simulink model "PMSM"  (Simulink 8.3)
settings: Solver=ode45  StartTime=0.0  StopTime=1  RelTol=1e-3
undefined symbols (not defined in the file): DiscIntNeverNeededParam
libraries: powerlib_meascontrol x9, powerlib x5
settings Model: Creator=JC  LastModifiedBy=JC
settings DataIOCC: SignalLoggingSaveFormat=Dataset
settings DebuggingCC: UnderspecifiedInitializationDetection=Simplified  StateNameClashWarn=none
settings GRTTargetCC: CombineOutputUpdateFcns=on  GRTInterface=off

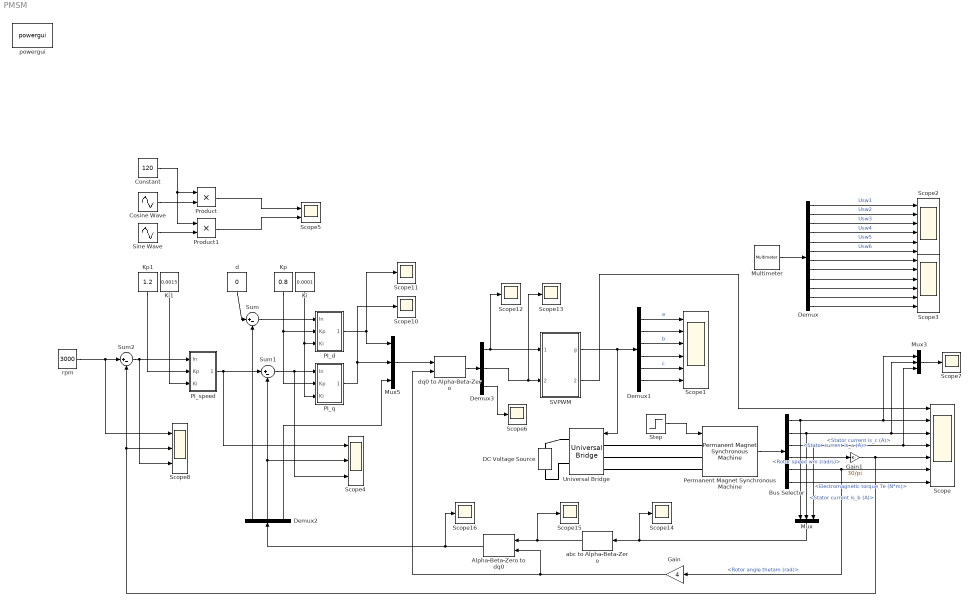
== system PMSM ==
  " Cosine Wave" : Sin  Frequency=pi*2/0.36  Phase=pi/2  Samples=360  SampleTime=0.001  Offset=90
  Alpha-Beta-Zero to dq0 : powerlib_meascontrol/Transformations/Alpha-Beta-Zero to dq0  Alignment=Aligned with phase A axis
  Bus Selector : BusSelector  OutputSignals=Stator current is_a (A),Stator current is_b (A),Stator current is_c (A),Rotor speed wm (rad/s),Rotor angle thetam (rad),Electromagnetic torque Te (N*m)
  Constant : Constant  Value=120
  DC Voltage Source : powerlib/Electrical Sources/DC Voltage Source  Amplitude=310  Measurements=None
  Demux : Demux  Outputs=12
  Demux1 : Demux  Outputs=6
  Demux2 : Demux  Outputs=3
  Demux3 : Demux  Outputs=3
  Gain : Gain  Gain=4
  Gain1 : Gain  Gain=30/pi
  Ki : Constant  Value=0.0001
  Ki1 : Constant  Value=0.0015
  Kp : Constant  Value=0.8
  Kp1 : Constant  Value=1.2
  Multimeter : powerlib/Measurements/Multimeter  PhasorSimulation=off  OutputType=Complex  sel=[1 2 3 4 5 6 11 12 13 14 15 16]  L=16  Gain=[1 1 1 1 1 1 1 1 1 1 1 1]  yselected={'Usw1: Universal Bridge','Usw2: Universal Bridge','Usw3: Universal Bridge','Usw4: Universal Bridge','Usw5: Universal Bridge','Usw6: Universal Bridge','Isw1: Universal Bridge','Isw2: Universal Bridge','Isw3: Universal Bridge','Isw4: Universal Bridge','Isw5: Universal Bridge','Isw6: Universal Bridge'};  PSBOutputType=1  PSBequivalent=0  AxesSetting=[0,0.1,-100,100]  Display=0  SavedBlockNames=-11
  Mux : Mux  Inputs=3
  Mux3 : Mux  Inputs=3
  Mux5 : Mux  Inputs=3
  PI_d : Subsystem
  PI_q : Subsystem
  PI_speed : Subsystem
  Permanent Magnet Synchronous Machine : powerlib/Machines/Permanent Magnet Synchronous Machine  NbPhases=3  FluxDistribution=Sinusoidal  RotorType=Round  MechanicalLoad=Torque Tm  PresetModel=No  ShowDetailedParameters=on  MeasurementBus=off  Resistance=3.3  Inductance=8.5e-3  dqInductances=[8.5e-3,8.5e-3]  La=0.00956  MachineConstant=Flux linkage established by magnets (V.s)  Flux=0.07147  VoltageCst=51.8529  TorqueCst=0.42882  Flat=120  Mechanical=[0.00062 0.0003035 4 0]  PolePairs=4  InitialConditions=[0,0, 0,0]  InitialConditions5ph=[0 0 0 0 0 0]  TsPowergui=0  TsBlock=-1  RefAngle=Aligned with phase A axis (original Park)
  Product : Product
  Product1 : Product
  SVPWM : Subsystem
  Scope : Scope  NumInputPorts=7
      settings: YMin=0~-5~-5~-5~-5~0~-5  YMax=8~5~5~5~5~10~5  SaveName=ScopeData2
  Scope1 : Scope  NumInputPorts=6
      settings: YMin=-5~-5~-5~-5~-5~-5  YMax=5~5~5~5~5~5  SaveName=ScopeData6
  Scope{6..7,10..16} (9 alike) : Scope
      Scope10 settings: SaveName=ScopeData15
      Scope11 settings: SaveName=ScopeData16
      Scope12 settings: SaveName=ScopeData17
      Scope13 settings: SaveName=ScopeData18
      Scope14 settings: SaveName=ScopeData19
      Scope15 settings: SaveName=ScopeData20
      Scope16 settings: SaveName=ScopeData21
      Scope6 settings: SaveName=ScopeData11
      Scope7 settings: SaveName=ScopeData12
  Scope2 : Scope  NumInputPorts=6
      settings: YMin=-5~-5~-5~-5~-5~-5  YMax=5~5~5~5~5~5
  Scope3 : Scope  NumInputPorts=6
      settings: YMin=-5~-5~-5~-5~-5~-5  YMax=5~5~5~5~5~5  SaveName=ScopeData8
  Scope4 : Scope  NumInputPorts=3
      settings: YMin=-5~-5~-5  YMax=5~5~5  SaveName=ScopeData9
  Scope5 : Scope  NumInputPorts=2
      settings: YMin=-5~-5  YMax=5~5  SaveName=ScopeData10
  Scope8 : Scope  NumInputPorts=3
      settings: YMin=-5~-5~-5  YMax=5~5~5  SaveName=ScopeData13
  Sine Wave : Sin  Frequency=pi*2/0.36  Samples=360  SampleTime=0.001
  Step : Step  Time=0  After=0  SampleTime=0
  Sum : Sum  Inputs=|+-
  Sum1 : Sum  Inputs=|+-
  Sum2 : Sum  Inputs=|+-
  Universal Bridge : powerlib/Power Electronics/Universal Bridge  Arms=3  SnubberResistance=1e5  SnubberCapacitance=inf  Device=IGBT / Diodes  Ron=1e-3  Lon=0  ForwardVoltages="[  0  0  ]"  ForwardVoltage=0  GTOparameters=[ 10e-6 , 20e-6 ]  IGBTparameters=[ 1e-6 , 2e-6 ]  Measurements=All voltages and currents  Measurements_2=None  converterType=Rectifier
  abc to Alpha-Beta-Zero : powerlib_meascontrol/Transformations/abc to Alpha-Beta-Zero
  d : Constant  Value=0
  dq0 to Alpha-Beta-Zero : powerlib_meascontrol/Transformations/dq0 to Alpha-Beta-Zero  Alignment=Aligned with phase A axis
  powergui : powerlib/powergui  RequirementInfo="{}  %GIDa_c9ce1342_5d33_47b2_941f_a20f6faa6b6c"  Priority=1  SimulationMode=Discrete  SolverType=Tustin  SampleTime=50e-6  frequency=60  SPID=off  DisableSnubberDevices=off  DisableRonSwitches=off  DisableVfSwitches=off  SwTol=0  Interpol=off  DisplayEquations=off  Ts=0  methode=off  frequencyindice=0  Pbase=100e6  ErrMax=1e-4  Iterations=50  UnitsV=kV  UnitsW=MW  FunctionMessages=off  echomessages=off  HookPort=off  EnableUseOfTLC=off  x0status=blocks  RestoreLinks=warning  ResistiveCurrentMeasurement=off  Frange=[0:2:500]  Ylog=off  Xlog=on  ShowGrid=off  save=off  variable=ZData  structure=0  ZoomFFT=off  StartTime=0.0  cycles=1  DisplayStyle=1  fundamental=60  FreqAxis=off  MaxFrequency=1000  frequencyindicesteady=1  RmsSteady=1  display=off
  rpm : Constant  Value=3000
  wires:
  Step/1 -> Permanent Magnet Synchronous Machine/1
  Bus Selector/2 -> Mux3/2, Scope/3, Mux/2  "<Stator current is_b (A)>"
  Bus Selector/3 -> Mux3/3, Scope/4, Mux/3  "<Stator current is_c (A)>"
  Bus Selector/4 -> Gain1/1  "<Rotor speed wm (rad/s)>"
  Bus Selector/5 -> Gain/1, Scope/6  "<Rotor angle thetam (rad)>"
  Bus Selector/6 -> Scope/7  "<Electromagnetic torque Te (N*m)>"
  Multimeter/1 -> Demux/1
  SVPWM/1(g) -> Demux1/1, Universal Bridge/1
  Demux1/1 -> Scope1/1  "a"
  Demux1/2 -> Scope1/2
  Demux1/3 -> Scope1/3  "b"
  Demux1/4 -> Scope1/4
  Demux1/5 -> Scope1/5  "c"
  Demux1/6 -> Scope1/6
  SVPWM/2(sector) -> Scope/1
  Bus Selector/1 -> Mux3/1, Scope/2, Mux/1  "<Stator current is_a (A)>"
  Permanent Magnet Synchronous Machine/1 -> Bus Selector/1
  abc to Alpha-Beta-Zero/1 -> Scope15/1, Alpha-Beta-Zero to dq0/1
  Constant/1 -> Product1/1, Product/1
  " Cosine Wave"/1 -> Product/2
  Sine Wave/1 -> Product1/2
  Product/1 -> Scope5/1
  Product1/1 -> Scope5/2
  dq0 to Alpha-Beta-Zero/1 -> Demux3/1
  Demux3/3 -> Scope6/1
  Demux3/1 -> SVPWM/1(Ualpha), Scope12/1
  Demux3/2 -> Scope13/1, SVPWM/2("Ubeta ")
  Mux3/1 -> Scope7/1
  Alpha-Beta-Zero to dq0/1 -> Scope16/1, Demux2/1
  Mux/1 -> Scope14/1, abc to Alpha-Beta-Zero/1
  Gain/1 -> dq0 to Alpha-Beta-Zero/2, Alpha-Beta-Zero to dq0/2
  Demux2/1 -> Sum/2
  Sum/1 -> PI_d/1(In)
  Demux2/2 -> Sum1/2, Scope4/2
  Sum1/1 -> Scope4/3, PI_q/1(In)
  PI_q/1("Out ") -> Mux5/2, Scope10/1
  PI_d/1("Out ") -> Scope11/1, Mux5/1
  Mux5/1 -> dq0 to Alpha-Beta-Zero/1
  d/1 -> Sum/1
  PI_speed/1("Out ") -> Scope4/1, Sum1/1
  Ki/1 -> PI_d/3(Ki), PI_q/3(Ki)
  Kp/1 -> PI_d/2(Kp), PI_q/2(Kp)
  Demux2/3 -> Mux5/3
  Gain1/1 -> Scope/5, Sum2/2, Scope8/2
  Ki1/1 -> PI_speed/3(Ki)
  Kp1/1 -> PI_speed/2(Kp)
  Sum2/1 -> Scope8/3, PI_speed/1(In)
  rpm/1 -> Scope8/1, Sum2/1
  Demux/1 -> Scope2/1  "Usw1"
  Demux/2 -> Scope2/2  "Usw2"
  Demux/3 -> Scope2/3  "Usw3"
  Demux/4 -> Scope2/4  "Usw4"
  Demux/5 -> Scope2/5  "Usw5"
  Demux/6 -> Scope2/6  "Usw6"
  Demux/7 -> Scope3/1
  Demux/8 -> Scope3/2
  Demux/9 -> Scope3/3
  Demux/10 -> Scope3/4
  Demux/11 -> Scope3/5
  Demux/12 -> Scope3/6
  connections:
  Universal Bridge/LConn1 -- Permanent Magnet Synchronous Machine/LConn1
  Universal Bridge/LConn2 -- Permanent Magnet Synchronous Machine/LConn2
  Universal Bridge/LConn3 -- Permanent Magnet Synchronous Machine/LConn3
  Universal Bridge/RConn1 -- DC Voltage Source/RConn1
  Universal Bridge/RConn2 -- DC Voltage Source/LConn1

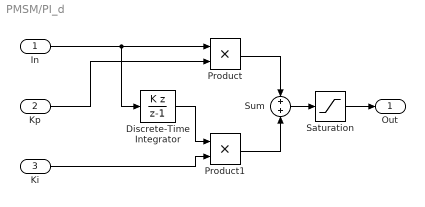
== system PMSM/PI_d ==
  In : Inport
  Kp : Inport  Port=2
  Ki : Inport  Port=3
  Discrete-Time Integrator : DiscreteIntegrator  IntegratorMethod=Accumulation: Backward Euler  SampleTime=0.0005  ICPrevOutput=DiscIntNeverNeededParam  ICPrevScaledInput=DiscIntNeverNeededParam
  Product : Product
  Product1 : Product
  Saturation : Saturate  UpperLimit=300  LowerLimit=-300
  Sum : Sum  Inputs=+|+
  "Out " : Outport
  wires:
  In/1 -> Discrete-Time Integrator/1, Product/1
  Kp/1 -> Product/2
  Discrete-Time Integrator/1 -> Product1/1
  Ki/1 -> Product1/2
  Product/1 -> Sum/1
  Product1/1 -> Sum/2
  Sum/1 -> Saturation/1
  Saturation/1 -> "Out "/1

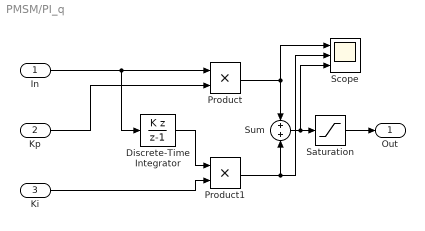
== system PMSM/PI_q ==
  In : Inport
  Kp : Inport  Port=2
  Ki : Inport  Port=3
  Discrete-Time Integrator : DiscreteIntegrator  IntegratorMethod=Accumulation: Backward Euler  SampleTime=0.0005  ICPrevOutput=DiscIntNeverNeededParam  ICPrevScaledInput=DiscIntNeverNeededParam
  Product : Product
  Product1 : Product
  Saturation : Saturate  UpperLimit=300  LowerLimit=-300
  Scope : Scope  NumInputPorts=3
      settings: YMin=-5~-5~-5  YMax=5~5~5  SaveName=ScopeData22
  Sum : Sum  Inputs=+|+
  "Out " : Outport
  wires:
  In/1 -> Discrete-Time Integrator/1, Product/1
  Kp/1 -> Product/2
  Discrete-Time Integrator/1 -> Product1/1
  Ki/1 -> Product1/2
  Product/1 -> Scope/1, Sum/1
  Product1/1 -> Sum/2, Scope/2
  Sum/1 -> Scope/3, Saturation/1
  Saturation/1 -> "Out "/1

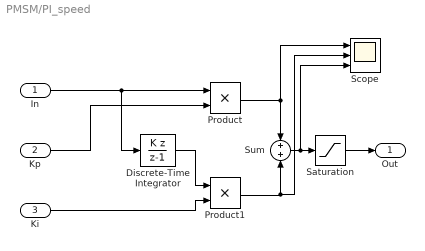
== system PMSM/PI_speed ==
  In : Inport
  Kp : Inport  Port=2
  Ki : Inport  Port=3
  Discrete-Time Integrator : DiscreteIntegrator  IntegratorMethod=Accumulation: Backward Euler  SampleTime=0.0005  ICPrevOutput=DiscIntNeverNeededParam  ICPrevScaledInput=DiscIntNeverNeededParam
  Product : Product
  Product1 : Product
  Saturation : Saturate  UpperLimit=4000  LowerLimit=-4000
  Scope : Scope  NumInputPorts=3
      settings: YMin=-5~-5~-5  YMax=5~5~5  SaveName=ScopeData14
  Sum : Sum  Inputs=+|+
  "Out " : Outport
  wires:
  In/1 -> Discrete-Time Integrator/1, Product/1
  Kp/1 -> Product/2
  Discrete-Time Integrator/1 -> Product1/1
  Ki/1 -> Product1/2
  Product/1 -> Sum/1, Scope/1
  Product1/1 -> Scope/2, Sum/2
  Sum/1 -> Scope/3, Saturation/1
  Saturation/1 -> "Out "/1

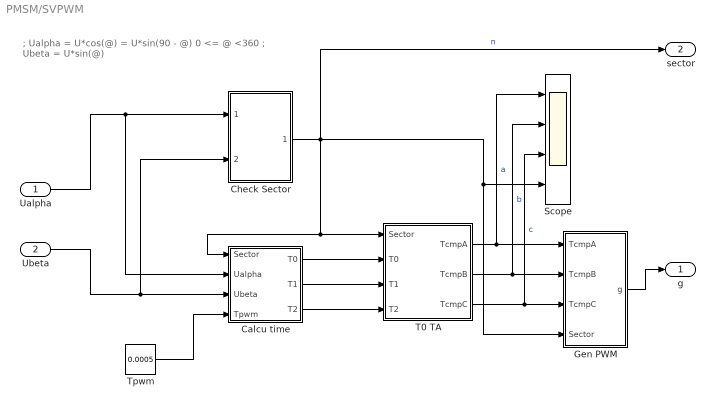
== system PMSM/SVPWM ==
  note: ; Ualpha = U*cos(@) = U*sin(90 - @)  0 <= @ <360
      | ; Ubeta  = U*sin(@)
  Ualpha : Inport
  "Ubeta " : Inport  Port=2
  Calcu time : Subsystem
  Check Sector : Subsystem
  "Gen PWM " : Subsystem
  Scope : Scope  NumInputPorts=4
      settings: YMin=-5~-5~-5~-5  YMax=5~5~5~5  SaveName=ScopeData5
  "T0 TA " : Subsystem
  Tpwm : Constant  Value=0.0005
  g : Outport
  sector : Outport  Port=2
  wires:
  "T0 TA "/1(TcmpA) -> "Gen PWM "/1(TcmpA), Scope/1  "a"
  "T0 TA "/2(TcmpB) -> Scope/2, "Gen PWM "/2(TcmpB)  "b"
  "T0 TA "/3(TcmpC) -> Scope/3, "Gen PWM "/3(TcmpC)  "c"
  Ualpha/1 -> Check Sector/1(Ualpha), Calcu time/2("Ualpha ")
  "Ubeta "/1 -> Check Sector/2(Ubeta), Calcu time/3(Ubeta)
  Check Sector/1(Sector) -> sector/1, Calcu time/1(Sector), "T0 TA "/1(Sector), "Gen PWM "/4(Sector), Scope/4  "n"
  Calcu time/1(T0) -> "T0 TA "/2(T0)
  Calcu time/2(T1) -> "T0 TA "/3(T1)
  Calcu time/3(T2) -> "T0 TA "/4(T2)
  "Gen PWM "/1(g) -> g/1
  Tpwm/1 -> Calcu time/4(Tpwm)

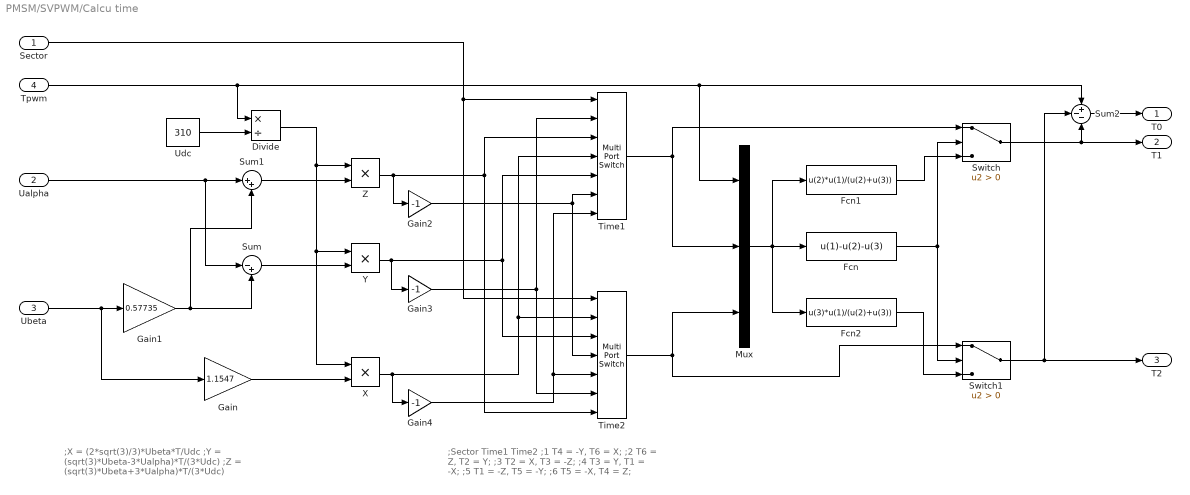
== system PMSM/SVPWM/Calcu time ==
  note: ;Sector	Time1	 Time2
      | ;1	T4 = -Y,	T6 =  X;
      | ;2	T6 =  Z,	T2 =  Y;
      | ;3	T2 =  X,	T3 = -Z;
      | ;4	T3 =  Y,	T1 = -X;
      | ;5	T1 = -Z,	T5 = -Y;
      | ;6	T5 = -X,	T4 =  Z;
  note: ;X = (2*sqrt(3)/3)*Ubeta*T/Udc
      | ;Y = (sqrt(3)*Ubeta-3*Ualpha)*T/(3*Udc)
      | ;Z = (sqrt(3)*Ubeta+3*Ualpha)*T/(3*Udc)
  Sector : Inport
  "Ualpha " : Inport  Port=2
  Ubeta : Inport  Port=3
  Tpwm : Inport  Port=4
  Divide : Product  Inputs=*/
  Fcn : Fcn  Expr=u(1)-u(2)-u(3)
  Fcn1 : Fcn  Expr=u(2)*u(1)/(u(2)+u(3))
  Fcn2 : Fcn  Expr=u(3)*u(1)/(u(2)+u(3))
  Gain : Gain  Gain=1.1547
  Gain1 : Gain  Gain=0.57735
  Gain2 : Gain  Gain=-1
  Gain3 : Gain  Gain=-1
  Gain4 : Gain  Gain=-1
  Mux : Mux  Inputs=3
  Sum : Sum  Inputs=|-+
  Sum1 : Sum  Inputs=|++
  Sum2 : Sum  Inputs=+--
  Switch : Switch  Criteria=u2 > Threshold
  Switch1 : Switch  Criteria=u2 > Threshold
  Time1 : MultiPortSwitch  Inputs=6
  Time2 : MultiPortSwitch  Inputs=6
  Udc : Constant  Value=310
  X : Product
  Y : Product
  Z : Product
  T0 : Outport
  T1 : Outport  Port=2
  T2 : Outport  Port=3
  wires:
  Sum1/1 -> Z/2
  Divide/1 -> X/1, Y/1, Z/1
  Tpwm/1 -> Divide/1, Sum2/1, Mux/1
  Sum/1 -> Y/2
  Gain2/1 -> Time2/4, Time1/6
  Fcn/1 -> Switch1/2, Switch/2
  Time2/1 -> Switch1/1, Mux/3
  Time1/1 -> Mux/2, Switch/1
  Mux/1 -> Fcn2/1, Fcn1/1, Fcn/1
  Y/1 -> Gain3/1, Time2/3, Time1/5
  Gain3/1 -> Time2/6, Time1/2
  Sector/1 -> Time1/1, Time2/1
  Z/1 -> Time1/3, Time2/7, Gain2/1
  Switch1/1 -> T2/1, Sum2/2
  Gain/1 -> X/2
  Switch/1 -> T1/1, Sum2/3
  Udc/1 -> Divide/2
  Gain4/1 -> Time1/7, Time2/5
  Fcn1/1 -> Switch/3
  X/1 -> Time2/2, Time1/4, Gain4/1
  Fcn2/1 -> Switch1/3
  Sum2/1 -> T0/1
  Gain1/1 -> Sum1/2, Sum/2
  Ubeta/1 -> Gain/1, Gain1/1
  "Ualpha "/1 -> Sum/1, Sum1/1

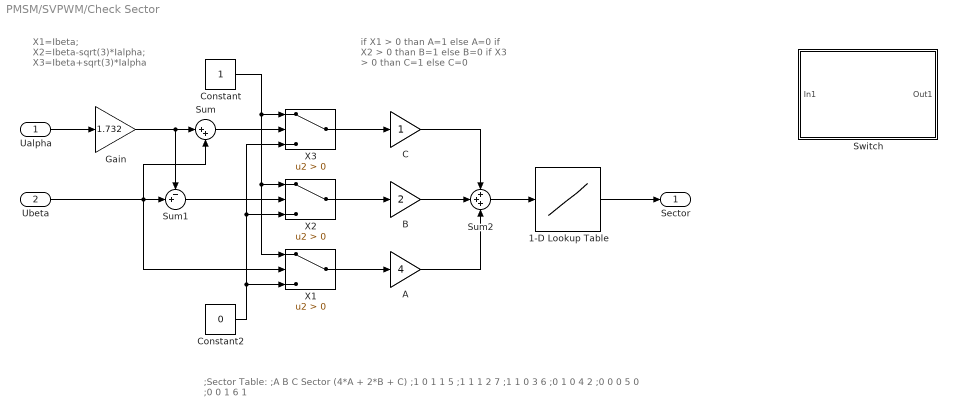
== system PMSM/SVPWM/Check Sector ==
  note: ;Sector Table:
      | ;A	B	C	Sector	(4*A + 2*B + C)
      | ;1	0	1	1	5
      | ;1	1	1	2	7
      | ;1	1	0	3	6
      | ;0	1	0	4	2
      | ;0	0	0	5	0
      | ;0	0	1	6	1
  note: if X1 > 0 than A=1 else A=0
      | if X2 > 0 than B=1 else B=0
      | if X3 > 0 than C=1 else C=0
  note: X1=Ibeta;
      | X2=Ibeta-sqrt(3)*Ialpha;
      | X3=Ibeta+sqrt(3)*Ialpha
  Ualpha : Inport
  Ubeta : Inport  Port=2
  1-D Lookup Table : Lookup_n-D  NumberOfTableDimensions=1  BreakpointsForDimension1=[0 1 2 5 6 7]  Table=[5 6 4 1 3 2]  InternalRulePriority=Speed  RndMeth=Simplest  InputSameDT=on
  A : Gain  Gain=4
  B : Gain  Gain=2
  C : Gain
  Constant : Constant
  Constant2 : Constant  Value=0
  Gain : Gain  Gain=1.732
  Sum : Sum  Inputs=|++
  Sum1 : Sum  Inputs=-+|
  Sum2 : Sum  Inputs=+++
  Switch : Subsystem
  X1 : Switch  Criteria=u2 > Threshold
  X2 : Switch  Criteria=u2 > Threshold
  X3 : Switch  Criteria=u2 > Threshold
  Sector : Outport
  wires:
  Ubeta/1 -> Sum1/2, X1/2, Sum/2
  Gain/1 -> Sum/1, Sum1/1
  Ualpha/1 -> Gain/1
  Sum/1 -> X3/2
  X2/1 -> B/1
  X3/1 -> C/1
  X1/1 -> A/1
  Sum1/1 -> X2/2
  Constant/1 -> X1/1, X2/1, X3/1
  Constant2/1 -> X3/3, X2/3, X1/3
  C/1 -> Sum2/1
  B/1 -> Sum2/2
  A/1 -> Sum2/3
  Sum2/1 -> 1-D Lookup Table/1
  1-D Lookup Table/1 -> Sector/1

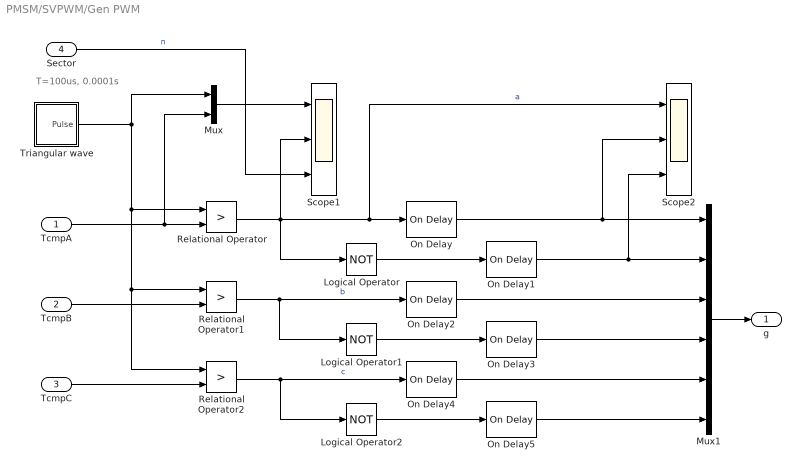
== system PMSM/SVPWM/Gen PWM  ==
  note: T=100us, 0.0001s
  TcmpA : Inport
  TcmpB : Inport  Port=2
  TcmpC : Inport  Port=3
  Sector : Inport  Port=4
  Logical Operator : Logic  Operator=NOT  AllPortsSameDT=off  OutDataTypeStr=boolean
  Logical Operator1 : Logic  Operator=NOT  AllPortsSameDT=off  OutDataTypeStr=boolean
  Logical Operator2 : Logic  Operator=NOT  AllPortsSameDT=off  OutDataTypeStr=boolean
  Mux : Mux  Inputs=2
  Mux1 : Mux  Inputs=6
  On Delay{,1..5} (6 alike) : powerlib_meascontrol/Logic/On Delay  DelayType=On delay  delay=0.000005  ic=0  Ts=0
  Relational Operator : RelationalOperator  Operator=>  OutDataTypeStr=boolean
  Relational Operator1 : RelationalOperator  Operator=>  OutDataTypeStr=boolean
  Relational Operator2 : RelationalOperator  Operator=>  OutDataTypeStr=boolean
  Scope1 : Scope  NumInputPorts=3
      settings: YMin=-5~-5~-5  YMax=5~5~5  SaveName=ScopeData3
  Scope2 : Scope  NumInputPorts=3
      settings: YMin=-5~-5~-5  YMax=5~5~5
  Triangular wave : Subsystem
  g : Outport
  wires:
  Triangular wave/1("Pulse ") -> Relational Operator2/1, Relational Operator1/1, Relational Operator/1, Mux/1
  TcmpA/1 -> Mux/2, Relational Operator/2
  Relational Operator/1 -> Scope1/2, Logical Operator/1, Scope2/1, On Delay/1  "a"
  TcmpB/1 -> Relational Operator1/2
  TcmpC/1 -> Relational Operator2/2
  Relational Operator2/1 -> Logical Operator2/1, On Delay4/1  "c"
  Relational Operator1/1 -> Logical Operator1/1, On Delay2/1  "b"
  Logical Operator2/1 -> On Delay5/1
  Logical Operator1/1 -> On Delay3/1
  Logical Operator/1 -> On Delay1/1
  Mux/1 -> Scope1/1
  Sector/1 -> Scope1/3  "n"
  Mux1/1 -> g/1
  On Delay/1 -> Scope2/2, Mux1/1
  On Delay1/1 -> Scope2/3, Mux1/2
  On Delay2/1 -> Mux1/3
  On Delay3/1 -> Mux1/4
  On Delay4/1 -> Mux1/5
  On Delay5/1 -> Mux1/6

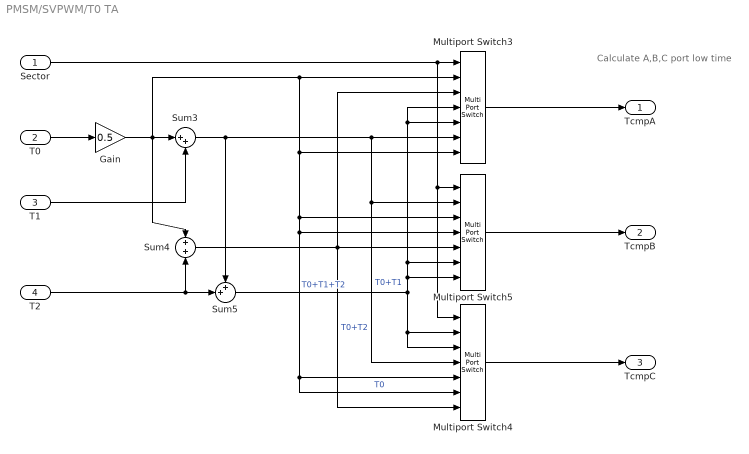
== system PMSM/SVPWM/T0 TA  ==
  note: Calculate A,B,C port low time
  Sector : Inport
  T0 : Inport  Port=2
  T1 : Inport  Port=3
  T2 : Inport  Port=4
  Gain : Gain  Gain=0.5
  Multiport Switch3 : MultiPortSwitch  Inputs=6
  Multiport Switch4 : MultiPortSwitch  Inputs=6
  Multiport Switch5 : MultiPortSwitch  Inputs=6
  Sum3 : Sum  Inputs=|++
  Sum4 : Sum  Inputs=+|+
  Sum5 : Sum  Inputs=++|
  TcmpA : Outport
  TcmpB : Outport  Port=2
  TcmpC : Outport  Port=3
  wires:
  Gain/1 -> Sum4/1, Multiport Switch3/2, Multiport Switch3/7, Multiport Switch4/6, Multiport Switch4/5, Multiport Switch5/4, Multiport Switch5/3, Sum3/1  "T0"
  Sector/1 -> Multiport Switch3/1, Multiport Switch4/1, Multiport Switch5/1
  T0/1 -> Gain/1
  Sum3/1 -> Sum5/1, Multiport Switch4/4, Multiport Switch5/2, Multiport Switch3/6  "T0+T1"
  Sum5/1 -> Multiport Switch5/7, Multiport Switch5/6, Multiport Switch3/5, Multiport Switch3/4, Multiport Switch4/2, Multiport Switch4/3  "T0+T1+T2"
  T1/1 -> Sum3/2
  T2/1 -> Sum5/2, Sum4/2
  Multiport Switch4/1 -> TcmpC/1
  Multiport Switch3/1 -> TcmpA/1
  Multiport Switch5/1 -> TcmpB/1
  Sum4/1 -> Multiport Switch4/7, Multiport Switch5/5, Multiport Switch3/3  "T0+T2"

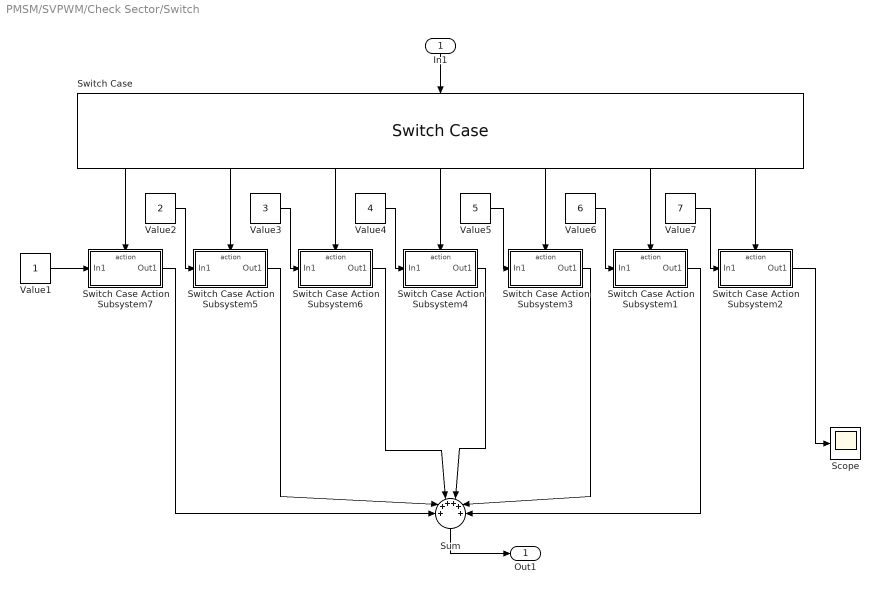
== system PMSM/SVPWM/Check Sector/Switch ==
  In1 : Inport
  Scope : Scope
      settings: SaveName=ScopeData7
  Sum : Sum  Inputs=++++++
  Switch Case : SwitchCase  CaseConditions={5,7,6,2,0,1}
  Switch Case Action Subsystem1 : Subsystem  TreatAsAtomicUnit=on
  Switch Case Action Subsystem2 : Subsystem  TreatAsAtomicUnit=on
  Switch Case Action Subsystem3 : Subsystem  TreatAsAtomicUnit=on
  Switch Case Action Subsystem4 : Subsystem  TreatAsAtomicUnit=on
  Switch Case Action Subsystem5 : Subsystem  TreatAsAtomicUnit=on
  Switch Case Action Subsystem6 : Subsystem  TreatAsAtomicUnit=on
  Switch Case Action Subsystem7 : Subsystem  TreatAsAtomicUnit=on
  Value1 : Constant
  Value2 : Constant  Value=2
  Value3 : Constant  Value=3
  Value4 : Constant  Value=4
  Value5 : Constant  Value=5
  Value6 : Constant  Value=6
  Value7 : Constant  Value=7
  Out1 : Outport
  wires:
  Switch Case Action Subsystem6/1(Out1) -> Sum/3
  Switch Case Action Subsystem3/1(Out1) -> Sum/5
  Switch Case Action Subsystem2/1(Out1) -> Scope/1
  Switch Case Action Subsystem5/1(Out1) -> Sum/2
  Switch Case Action Subsystem1/1(Out1) -> Sum/6
  Switch Case Action Subsystem4/1(Out1) -> Sum/4
  Value6/1 -> Switch Case Action Subsystem1/1(In1)
  Switch Case/5 -> Switch Case Action Subsystem3/Action
  Value1/1 -> Switch Case Action Subsystem7/1(In1)
  Switch Case/3 -> Switch Case Action Subsystem6/Action
  Switch Case/1 -> Switch Case Action Subsystem7/Action
  Switch Case/2 -> Switch Case Action Subsystem5/Action
  Switch Case Action Subsystem7/1(Out1) -> Sum/1
  Switch Case/7 -> Switch Case Action Subsystem2/Action
  Value3/1 -> Switch Case Action Subsystem6/1(In1)
  Value5/1 -> Switch Case Action Subsystem3/1(In1)
  Value7/1 -> Switch Case Action Subsystem2/1(In1)
  Value4/1 -> Switch Case Action Subsystem4/1(In1)
  Switch Case/4 -> Switch Case Action Subsystem4/Action
  Value2/1 -> Switch Case Action Subsystem5/1(In1)
  Switch Case/6 -> Switch Case Action Subsystem1/Action
  Sum/1 -> Out1/1
  In1/1 -> Switch Case/1

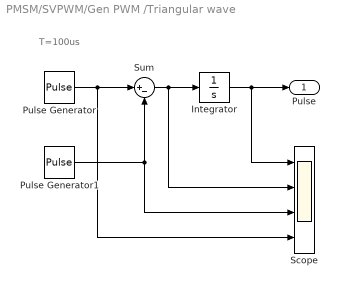
== system PMSM/SVPWM/Gen PWM /Triangular wave ==
  note: T=100us
  Integrator : Integrator
  Pulse Generator : DiscretePulseGenerator  PulseType=Time based  Amplitude=2  Period=0.0005  PulseWidth=50
  Pulse Generator1 : DiscretePulseGenerator  PulseType=Time based  Amplitude=2  Period=0.0005  PulseWidth=50  PhaseDelay=0.00025
  Scope : Scope  NumInputPorts=4
      settings: YMin=-5~-5~-5~-5  YMax=5~5~5~5  SaveName=ScopeData4
  Sum : Sum  Inputs=|+-
  "Pulse " : Outport
  wires:
  Sum/1 -> Scope/2, Integrator/1
  Pulse Generator1/1 -> Scope/3, Sum/2
  Pulse Generator/1 -> Scope/4, Sum/1
  Integrator/1 -> Scope/1, "Pulse "/1

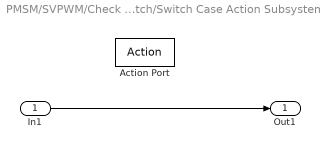
== system PMSM/SVPWM/Check Sector/Switch/Switch Case Action Subsystem1 ==
  In1 : Inport
  Action Port : ActionPort  ActionType=case
  Out1 : Outport
  wires:
  In1/1 -> Out1/1

== system PMSM/SVPWM/Check Sector/Switch/Switch Case Action Subsystem2 ==
  In1 : Inport
  Action Port : ActionPort  ActionType=default
  Out1 : Outport
  wires:
  In1/1 -> Out1/1

== system PMSM/SVPWM/Check Sector/Switch/Switch Case Action Subsystem3 ==
  In1 : Inport
  Action Port : ActionPort  ActionType=case
  Out1 : Outport
  wires:
  In1/1 -> Out1/1

== system PMSM/SVPWM/Check Sector/Switch/Switch Case Action Subsystem4 ==
  In1 : Inport
  Action Port : ActionPort  ActionType=case
  Out1 : Outport
  wires:
  In1/1 -> Out1/1

== system PMSM/SVPWM/Check Sector/Switch/Switch Case Action Subsystem5 ==
  In1 : Inport
  Action Port : ActionPort  ActionType=case
  Out1 : Outport
  wires:
  In1/1 -> Out1/1

== system PMSM/SVPWM/Check Sector/Switch/Switch Case Action Subsystem6 ==
  In1 : Inport
  Action Port : ActionPort  ActionType=case
  Out1 : Outport
  wires:
  In1/1 -> Out1/1

== system PMSM/SVPWM/Check Sector/Switch/Switch Case Action Subsystem7 ==
  In1 : Inport
  Action Port : ActionPort  ActionType=case
  Out1 : Outport
  wires:
  In1/1 -> Out1/1
